simulink model "TopLevel_Turbofan_DT_Faults"  (R2025a)
settings: Solver=ode15s  StartTime=0.0  StopTime=500  MaxStep=0.01  RelTol=1e-3
undefined symbols (not defined in the file or in its folder): BPR_design, DoUpgrade, Eff_hpt_map, Eff_Mod_Fan, Eff_Mod_HPC, Eff_Mod_HPC_Up, Eff_Mod_HPT, Eff_Mod_HPT_Up, Eff_Mod_LPC, Eff_Mod_LPC_Up, Eff_Mod_LPT, eta_hpc_map, eta_lpc_map, eta_lpt_map, Fan_eta_data, Fan_PR_data, FaultMode, flow_vec_fan, norm_flow_hpt, norm_speed_hpt, PR_hpc_map, PR_lpc_map, PR_lpt_map, speed_vec_fan, speed_vec_hpc, speed_vec_lpc, speed_vec_lpt, Torque_hpt_map, Wc_hpc_bp, Wc_lpc_bp, Wc_lpt_bp
libraries: fl_lib x10, nesl_utility x10, simulink x2, sdl_lib x2
(part 1 of 2)
settings Model: Creator=ramch  LastModifiedBy=ramch
settings DataIOCC: SaveFormat=StructureWithTime  SaveOutput=off  SaveState=on  DSMLogging=off  SaveTime=off  ReturnWorkspaceOutputs=off
settings SimscapeCC: SimscapeLogType=all  SimscapeLogSimulationStatistics=on  SimscapeLogToSDI=on  SimscapeLogOpenViewer=on  SimscapeLogName=simlog_TopLevel_Turbofan_DT_PDM  SimscapeLogLimitData=off

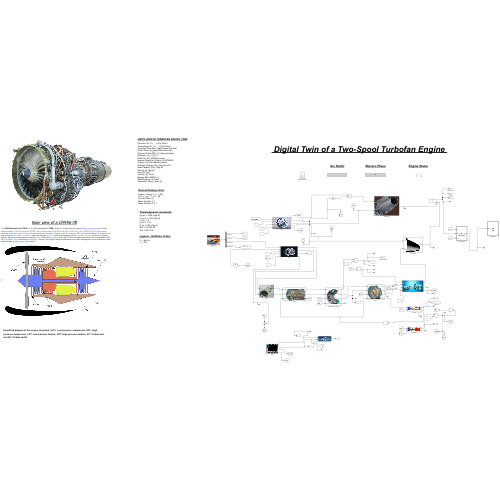
[thumbnail: Simulink's stored preview of the top-level diagram]
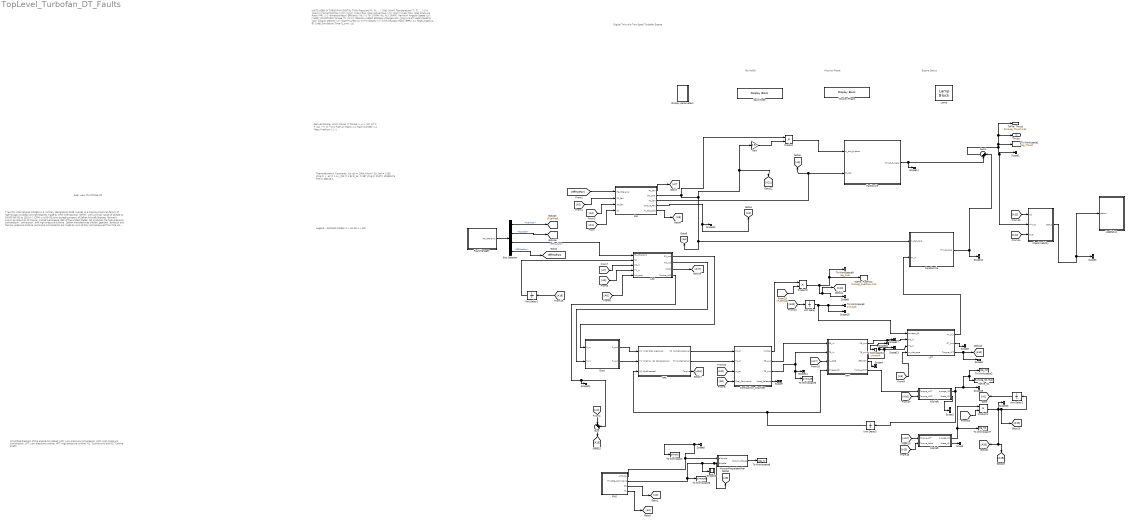
== system TopLevel_Turbofan_DT_Faults ==
  note: UNITS USED IN TURBOFAN DIGITAL TWIN
      | Pressure (P₀, P₁, …): [Pa] (N/m²)
      | Temperature (T₀, T₁, …): [K] (Kelvin)
      | Corrected Flow (Wc): [kg/s] (mass flow rate)
      | Actual Flow (ṁ): [kg/s] (mass flow rate)
      | Pressure Ratio (PR): [–] (dimensionless)
      | Efficiency (η): [–] (0–1)
      | RPM (N₁, N₂): [RPM] (rev/min)
      | Angular Speed (ω): [rad/s] (2π·RPM/60)
      | Torque (τ): [N·m] (Newton-meter)
      | Enthalpy Change (Δh): [J/kg] (cp·ΔT)
      | Heat Capacity (Cp): [J/kg·K]
      | Density (ρ): [kg/m³]
      | Area (A): [m²]
      | Velocity (V): [m/s]
      | Bypass Ratio (BPR): [–]
      | Shaft Angle (φ, θ): [rad]
      | Simulation Time (t_sim): [s]
  note: Digital Twin of a Two-Spool Turbofan Engine
  note: Engine Status
  note: Simplified diagram of the engine simulated (LPC: Low pressure compressor, HPC: High pressure compressor, LPT: Low pressure turbine, HPT: High pressure turbine, N1: Turbine axis and N2: Turbine shaft).
  note: T he CFM International CFM56 (U.S. military designation F108 ) series is a Franco-American family of high-bypass turbofan aircraft engines made by CFM International (CFMI), with a thrust range of 18,500 to 34,000 lbf (82 to 150 kN ). CFMI is a 50–50 joint-owned company of Safran Aircraft Engines (formerly known as Snecma) of France, and GE Aerospace (GE) of the United States. GE produces the high-pressure compressor , combustor , and high-pressure turbine , Safran manufactures the fan, gearbox , exhaust and the low-pressure turbine, and some components are made by Avio of Italy and Honeywell from the US. Both companies have their own final assembly line, GE in Evendale, Ohio , and Safran in Villaroche , France. The engine initially had extremely slow sales but has gone on to become the most used turbofan aircraft engine in the world.
  note: Legend – Go/NoGo Codes:
      |
      | 0 → No Go
      | 1 → GO
  note: Rear view of a CFM56-7B
  note: Derived Display Units:
      | Power = Torque × ω → [W]
      | ΔT = T_out − T_in → [K]
      | Fuel-Air Ratio: [–]
      | Mach Number: [–]
      | Mass Fraction X: [–]
  note: Go/ NoGO
  note: Thermodynamic Constants:
      | Cp_air = 1004 J/(kg·K)
      | Cp_hot = 1150 J/(kg·K)
      | γ_air = 1.4
      | γ_hot = 1.33
      | R_air = 287 J/(kg·K)
      | Pref = 101325 Pa
      | Tref = 288.15 K
  note: Mission Phase
  Bus Selector : BusSelector  OutputSignals=FuelMod,N1Scale,EffModLPC,EffModFan
  CheckViability : MATLAB Function  TreatAsAtomicUnit=on
  Combustion_Chamber : Subsystem
      mask Display: image('CC.jpg');
  CoreNozzle : Subsystem
      mask Display: image('CN.jpg');
  Display parameters : Subsystem
  Duct : Subsystem
      mask Display: image('Duct.jpg');
  FMS : Subsystem
      mask Display: image('FMS.jpg');
  Fan : Subsystem
      mask Display: image('Fan.jpg');
  FanNozzle : Subsystem
      mask Display: image('FN.jpg');
  FaultManager : Subsystem
      mask Display: image('Fault.jpg');
  Gain : Gain  Gain=5.5
  HPC : Subsystem
      mask Display: image('HPC.jpg');
  HPT : Subsystem
      mask Display: image('HPT.jpg');
  LPC : Subsystem
      mask Display: image('LPC.png');
  LPT : Subsystem
      mask Display: image('LPT.jpg');
  Lamp : LampBlock  LabelPosition=Hide  DefaultColor=[192.0, 192.0, 192.0]  Icon=CheckEngine
  LogStatus : MATLAB Function  TreatAsAtomicUnit=on
  Mission Phase : DisplayBlock  LabelPosition=Hide  Transparency=1  GridColor=[0.502, 0.502, 0.502]
  MissionPhaseIdentifier : Subsystem
      mask Display: image('Mission.jpg');
  N1shaft : Subsystem
      mask Display: image('shaft.jpg');
  N2shaft : Subsystem
      mask Display: image('shaft.jpg');
  Product : Product
  Product1 : Product
  Product2 : Product
  Scope{,1..21} (22 alike) : Scope
      Scope settings: ActiveDisplayYMinimum=-1  ActiveDisplayYMaximum=1
      Scope1 settings: ActiveDisplayYMinimum=-1  ActiveDisplayYMaximum=1
      Scope10 settings: ActiveDisplayYMinimum=-0.45859345963387366  ActiveDisplayYMaximum=1.635778226221027  DataLoggingVariableName=ScopeData10
      Scope11 settings: ActiveDisplayYMinimum=-1  ActiveDisplayYMaximum=1  DataLoggingVariableName=ScopeData11
      Scope12 settings: ActiveDisplayYMinimum=-1  ActiveDisplayYMaximum=1  DataLoggingVariableName=ScopeData12
      Scope13 settings: ActiveDisplayYMinimum=-609.11434420859632  ActiveDisplayYMaximum=1781.0190470175871  DataLoggingVariableName=ScopeData13
      Scope14 settings: ActiveDisplayYMinimum=-1  ActiveDisplayYMaximum=1  DataLoggingVariableName=ScopeData14
      Scope15 settings: ActiveDisplayYMinimum=-1  ActiveDisplayYMaximum=1  DataLoggingVariableName=ScopeData15
      Scope16 settings: ActiveDisplayYMinimum=-4.3963021341582635  ActiveDisplayYMaximum=4.6281003390981308  DataLoggingVariableName=ScopeData16
      Scope17 settings: ActiveDisplayYMinimum=-2.2429279816897957E+23  ActiveDisplayYMaximum=2.0186351835208165E+24  DataLoggingVariableName=ScopeData17
      Scope18 settings: ActiveDisplayYMinimum=-513.71209028734575  ActiveDisplayYMaximum=1737.7811833983071  DataLoggingVariableName=ScopeData18
      Scope19 settings: ActiveDisplayYMinimum=-0.12499999999999997  ActiveDisplayYMaximum=1.125  DataLoggingVariableName=ScopeData19
      Scope2 settings: ActiveDisplayYMinimum=-1  ActiveDisplayYMaximum=1  DataLoggingVariableName=ScopeData2
      Scope20 settings: ActiveDisplayYMinimum=-3.6198875871994079E+21  ActiveDisplayYMaximum=5.5031192284267649E+20  DataLoggingVariableName=ScopeData20
      Scope21 settings: ActiveDisplayYMinimum=-0.23453341351778778  ActiveDisplayYMaximum=0.2421108240195578  DataLoggingVariableName=ScopeData21
      Scope3 settings: ActiveDisplayYMinimum=-1  ActiveDisplayYMaximum=1  DataLoggingVariableName=ScopeData3
      Scope4 settings: ActiveDisplayYMinimum=-1.4197628335321743E+18  ActiveDisplayYMaximum=1.5775142594801933E+17  DataLoggingVariableName=ScopeData4
      Scope5 settings: ActiveDisplayYMinimum=-5201.9747686683695  ActiveDisplayYMaximum=12688.378863465885  DataLoggingVariableName=ScopeData5
      Scope6 settings: ActiveDisplayYMinimum=-1  ActiveDisplayYMaximum=1  DataLoggingVariableName=ScopeData6
      Scope7 settings: ActiveDisplayYMinimum=952444.62242727727  ActiveDisplayYMaximum=9.2631053030945715E+6  DataLoggingVariableName=ScopeData7
      Scope8 settings: ActiveDisplayYMinimum=-1  ActiveDisplayYMaximum=1  DataLoggingVariableName=ScopeData8
      Scope9 settings: ActiveDisplayYMinimum=-1  ActiveDisplayYMaximum=1  DataLoggingVariableName=ScopeData9
  Sum : Sum  Inputs=|++
  Sum1 : Sum  Inputs=|++
  To Workspace : ToWorkspace  VariableName=simout  SaveFormat=Timeseries  SampleTime=-1
  To Workspace1 : ToWorkspace  VariableName=log_Thrust  SaveFormat=Timeseries  SampleTime=-1
  To Workspace2 : ToWorkspace  VariableName=log_N2  SaveFormat=Timeseries  SampleTime=-1
  To Workspace3 : ToWorkspace  VariableName=simout3  SaveFormat=Timeseries  SampleTime=-1
  To Workspace4 : ToWorkspace  VariableName=simout4  SaveFormat=Timeseries  SampleTime=-1
  To Workspace5 : ToWorkspace  VariableName=simout5  SaveFormat=Timeseries  SampleTime=-1
  To Workspace6 : ToWorkspace  VariableName=simout6  SaveFormat=Timeseries  SampleTime=-1
  To Workspace7 : ToWorkspace  VariableName=log_N1  SaveFormat=Timeseries  SampleTime=-1
  To Workspace8 : ToWorkspace  VariableName=log_N  SaveFormat=Timeseries  SampleTime=-1
  To Workspace9 : ToWorkspace  VariableName=log_Fuel  SaveFormat=Timeseries  SampleTime=-1
  ToFile_FuelFlow : ToFile  Filename=RunLog_FuelFlow.mat  MatrixName=m_fuel  SaveFormat=Timeseries
  ToFile_N1 : ToFile  Filename=RunLog_N1.mat  MatrixName=omega_N1
  ToFile_Thrust : ToFile  Filename=RunLog_Thrust.mat  MatrixName=Thrust
  Unit Delay{,1..3} (4 alike) : UnitDelay  InitialCondition=1  SampleTime=-1  HasFrameUpgradeWarning=on
  fault Mode : DisplayBlock  LabelPosition=Hide  Transparency=1  GridColor=[0.502, 0.502, 0.502]
  Thrust : Outport
  wires:
  N2shaft/2(theta_N2) -> Scope1/1
  FaultManager/1(FaultParams) -> Bus Selector/1
  [A7] -> LPC/3(P2_in)
  Product1/1 -> [A20], [A18], [A13], Unit Delay2/1, Scope16/1
  HPC/1(P2 (outlet pressure)) -> Combustion_Chamber/1(P4_in)
  Fan/3(T1_fan) -> [A5], FanNozzle/2(T1_fan)
  CoreNozzle/1(Thrust_core) -> Scope12/1, Sum1/1
  Product2/1 -> To Workspace9/1, ToFile_FuelFlow/1, Scope8/1, [A14]
  Bus Selector/3 -> LPC/1(FaultParams)  "<EffModLPC>"
  Product/1 -> FanNozzle/1(m_dot_bypass)
  LPC/1(P3_out) -> Duct/1(P_in)
  Duct/2(T_out) -> HPC/2("T1 (inlet total temperature) ")
  Bus Selector/4 -> [EffModFan]  "<EffModFan>"
  [A6] -> LPC/5(Wc_core)
  [A4] -> Sum/1
  LPC/2(T3_out) -> Duct/2(T_in)
  HPC/2(T2 (outlet temp)) -> Combustion_Chamber/2(T4_in)
  LPC/4(Torque_LPC) -> Sum/2, Scope21/1
  N2shaft/1(omega_N2) -> To Workspace2/1, ToFile_N1/1, Scope15/1, Unit Delay3/1
  [EffModFan] -> Fan/1(FaultParams)
  Gain/1 -> Product/2
  [A2] -> Fan/2(P0_fan)
  [A3] -> Fan/3(T0_fan)
  [A1] -> Fan/4(N1)
  Duct/1(P_out) -> HPC/1(P1 (inlet total pressure))
  HPT/2(T6_out) -> Scope18/1, To Workspace4/1, Scope13/1, LPT/3(T6_in)
  Fan/1(" P1_fan") -> [A7]
  Fan/5(m_dot_core) -> [A9]
  HPT/1(P6_out) -> LPT/2(P6_in), Scope17/1
  FMS/1(Altitude) -> To Workspace/1, Scope5/1, MissionPhaseIdentifier/1(altitude)
  FMS/2(Throttle_Command) -> [A8], MissionPhaseIdentifier/2(throttle), Scope10/1, To Workspace6/1
  FMS/3(P0) -> [A2]
  FMS/4(T0) -> [A3]
  LPT/3(Torque_LPT) -> Scope9/1, [A10]
  Combustion_Chamber/2(P5_out) -> HPT/1(P5_in)
  Unit Delay3/1 -> HPC/3(N2 (shaft speed)), HPT/4(omega_N2)
  Combustion_Chamber/4(Heat_Release) -> Scope7/1
  Combustion_Chamber/3(T5_out) -> HPT/2(T5_in), To Workspace5/1, Scope14/1
  Combustion_Chamber/1(m_fuel) -> Product2/1
  MissionPhaseIdentifier/1(Mission_Phase) -> To Workspace8/1
  Unit Delay/1 -> Scope19/1, To Workspace3/1, LPT/1(omega_N1)
  Sum1/1 -> ToFile_Thrust/1, Thrust/1, To Workspace1/1, CheckViability/2(Thrust), Scope2/1
  HPT/4(Torque_HPT) -> N2shaft/1(Torque_HPT)
  FanNozzle/1(Thrust_bypass) -> Sum1/2, Scope11/1
  HPT/3(Eff_HPT) -> Scope4/1
  [A9] -> LPT/4(m_dot_core)
  LPT/2(P7_out) -> Scope6/1
  LPT/1(T7_out) -> CoreNozzle/2(T7_in)
  Unit Delay2/1 -> [A1]
  N1shaft/1(omega_N1) -> Product1/1, To Workspace7/1
  N1shaft/2(theta_N1) -> Scope/1
  CheckViability/1(status) -> Scope3/1, LogStatus/1(status)
  Fan/4(Torque_Fan) -> [A4], Scope20/1
  Fan/2(Wc_core) -> CoreNozzle/1(m_dot_core), [A6], [A21], Gain/1, Product/1
  [A13] -> CheckViability/1(N1)
  [A14] -> CheckViability/3(Fuel)
  Sum/1 -> [A15]
  [A15] -> N1shaft/2(Torque_Load)
  Bus Selector/2 -> [N1Scale]  "<N1Scale>"
  [N1Scale] -> Product1/2
  HPC/3(Torque) -> [A16]
  [A16] -> N2shaft/2(Torque_HPC)
  LPC/3(mdot) -> [A17]
  [A17] -> HPT/3(m_dot5)
  [A18] -> Unit Delay1/1
  Unit Delay1/1 -> LPC/2(N1)
  [A20] -> Unit Delay/1
  [A21] -> Combustion_Chamber/3(m_air)
  Bus Selector/1 -> [FuelMod]  "<FuelMod>"
  [FuelMod] -> Product2/2
  [A5] -> LPC/4(T2_in)
  [A8] -> Combustion_Chamber/4(Fuel_Command)
  [A10] -> N1shaft/1(Torque_LPT)

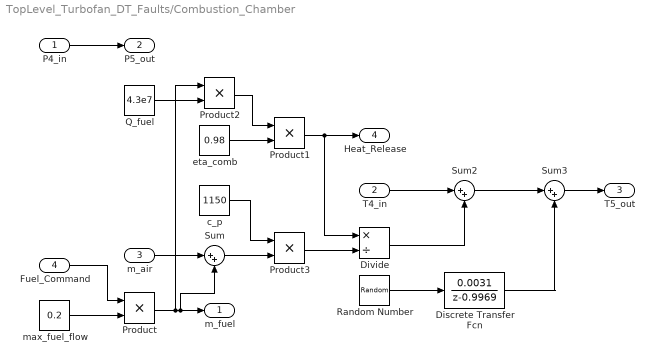
== system TopLevel_Turbofan_DT_Faults/Combustion_Chamber ==
  P4_in : Inport
  T4_in : Inport  Port=2
  m_air : Inport  Port=3
  Fuel_Command : Inport  Port=4
  Discrete Transfer Fcn : DiscreteTransferFcn  Numerator=0.0031  Denominator=1 -0.9969  InitialStates=0.001
  Divide : Product  Inputs=*/
  Product{,1..3} (4 alike) : Product
  Q_fuel : Constant  Value=4.3e7
  Random Number : RandomNumber  Variance=0.5  SampleTime=0.001
  Sum : Sum  Inputs=|++
  Sum2 : Sum  Inputs=|++
  Sum3 : Sum  Inputs=|++
  c_p : Constant  Value=1150
  eta_comb : Constant  Value=0.98
  max_fuel_flow : Constant  Value=0.2
  m_fuel : Outport
  P5_out : Outport  Port=2
  T5_out : Outport  Port=3
  Heat_Release : Outport  Port=4
  wires:
  T4_in/1 -> Sum2/1
  P4_in/1 -> P5_out/1
  Fuel_Command/1 -> Product/1
  m_air/1 -> Sum/1
  Sum3/1 -> T5_out/1
  Sum2/1 -> Sum3/1
  Sum/1 -> Product3/2
  eta_comb/1 -> Product1/2
  c_p/1 -> Product3/1
  max_fuel_flow/1 -> Product/2
  Random Number/1 -> Discrete Transfer Fcn/1
  Product3/1 -> Divide/2
  Product1/1 -> Divide/1, Heat_Release/1
  Product2/1 -> Product1/1
  Q_fuel/1 -> Product2/2
  Divide/1 -> Sum2/2
  Product/1 -> Sum/2, m_fuel/1, Product2/1
  Discrete Transfer Fcn/1 -> Sum3/2

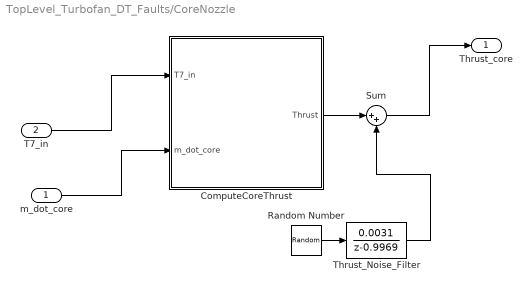
== system TopLevel_Turbofan_DT_Faults/CoreNozzle ==
  m_dot_core : Inport
  T7_in : Inport  Port=2
  ComputeCoreThrust : MATLAB Function  TreatAsAtomicUnit=on
  Random Number : RandomNumber  Variance=500  SampleTime=0.001
  Sum : Sum  Inputs=|++
  Thrust_Noise_Filter : DiscreteTransferFcn  Numerator=0.0031  Denominator=1 -0.9969  InitialStates=0.001
  Thrust_core : Outport
  wires:
  Sum/1 -> Thrust_core/1
  T7_in/1 -> ComputeCoreThrust/1(T7_in)
  Random Number/1 -> Thrust_Noise_Filter/1
  m_dot_core/1 -> ComputeCoreThrust/2(m_dot_core)
  ComputeCoreThrust/1(Thrust) -> Sum/1
  Thrust_Noise_Filter/1 -> Sum/2

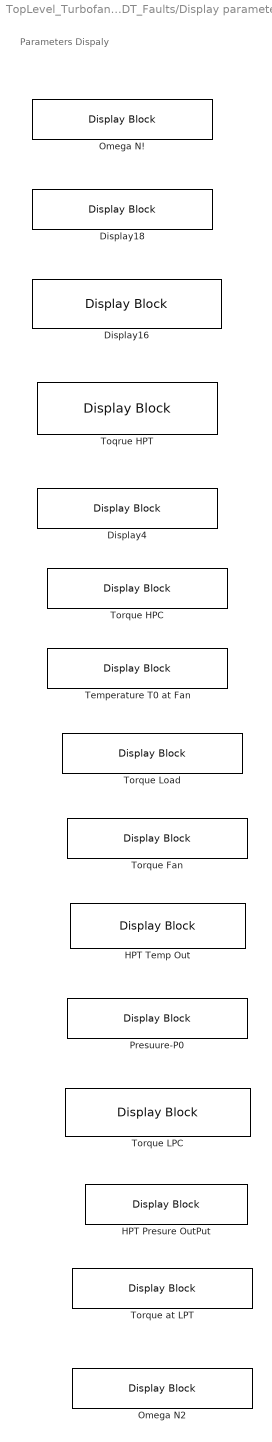
== system TopLevel_Turbofan_DT_Faults/Display parameters ==
  note: Parameters Dispaly
  Display16 : DisplayBlock  LabelPosition=Hide  Transparency=1  GridColor=[0.502, 0.502, 0.502]
  Display18 : DisplayBlock  LabelPosition=Hide  Transparency=1  GridColor=[0.502, 0.502, 0.502]
  Display4 : DisplayBlock  LabelPosition=Hide  Transparency=1  GridColor=[0.502, 0.502, 0.502]
  HPT Presure OutPut : DisplayBlock  LabelPosition=Hide  Transparency=1  GridColor=[0.502, 0.502, 0.502]
  HPT Temp Out : DisplayBlock  LabelPosition=Hide  Transparency=1  GridColor=[0.502, 0.502, 0.502]
  Omega N! : DisplayBlock  LabelPosition=Hide  Transparency=1  GridColor=[0.502, 0.502, 0.502]
  Omega N2 : DisplayBlock  LabelPosition=Hide  Transparency=1  GridColor=[0.502, 0.502, 0.502]
  Presuure-P0 : DisplayBlock  LabelPosition=Hide  Transparency=1  GridColor=[0.502, 0.502, 0.502]
  Temperature T0 at Fan : DisplayBlock  LabelPosition=Hide  Transparency=1  GridColor=[0.502, 0.502, 0.502]
  Toqrue HPT : DisplayBlock  LabelPosition=Hide  Transparency=1  GridColor=[0.502, 0.502, 0.502]
  Torque Fan : DisplayBlock  LabelPosition=Hide  Transparency=1  GridColor=[0.502, 0.502, 0.502]
  Torque HPC : DisplayBlock  LabelPosition=Hide  Transparency=1  GridColor=[0.502, 0.502, 0.502]
  Torque LPC : DisplayBlock  LabelPosition=Hide  Transparency=1  GridColor=[0.502, 0.502, 0.502]
  Torque Load : DisplayBlock  LabelPosition=Hide  Transparency=1  GridColor=[0.502, 0.502, 0.502]
  Torque at LPT : DisplayBlock  LabelPosition=Hide  Transparency=1  GridColor=[0.502, 0.502, 0.502]

== system TopLevel_Turbofan_DT_Faults/Duct ==
  P_in : Inport
  T_in : Inport  Port=2
  Gain : Gain  Gain=0.98
  P_out : Outport
  T_out : Outport  Port=2
  wires:
  Gain/1 -> P_out/1
  T_in/1 -> T_out/1
  P_in/1 -> Gain/1

== system TopLevel_Turbofan_DT_Faults/FMS ==
  Altitude_Profile : simulink/Sources/Repeating Sequence Interpolated  OutValues=[0 1500 6000 10000 10000 5000 0]  TimeValues=[0 50 100 200 300 400 500]  LookUpMeth=Interpolation-Use End Values  tsamp=0.1  OutMin=[]  OutMax=[]  OutDataTypeStr=double  OutputDataTypeScalingMode=double  OutDataType=fixdt(0,8)  OutScaling=2^-10
  AtmosphereModel : MATLAB Function  TreatAsAtomicUnit=on
  Throttle_Command_Profile : simulink/Sources/Repeating Sequence Interpolated  OutValues=[1.0 0.9 0.7 0.5 0.5 0.6 0.3]  TimeValues=[0 50 100 200 300 400 500]  LookUpMeth=Use Input Below  tsamp=0.1  OutMin=[]  OutMax=[]  OutDataTypeStr=double  OutputDataTypeScalingMode=double  OutDataType=fixdt(0,8)  OutScaling=2^-10
  Altitude : Outport
  Throttle_Command : Outport  Port=2
  P0 : Outport  Port=3
  T0 : Outport  Port=4
  wires:
  AtmosphereModel/1(P0) -> P0/1
  AtmosphereModel/2(T0) -> T0/1
  Altitude_Profile/1 -> AtmosphereModel/1(Altitude), Altitude/1
  Throttle_Command_Profile/1 -> Throttle_Command/1

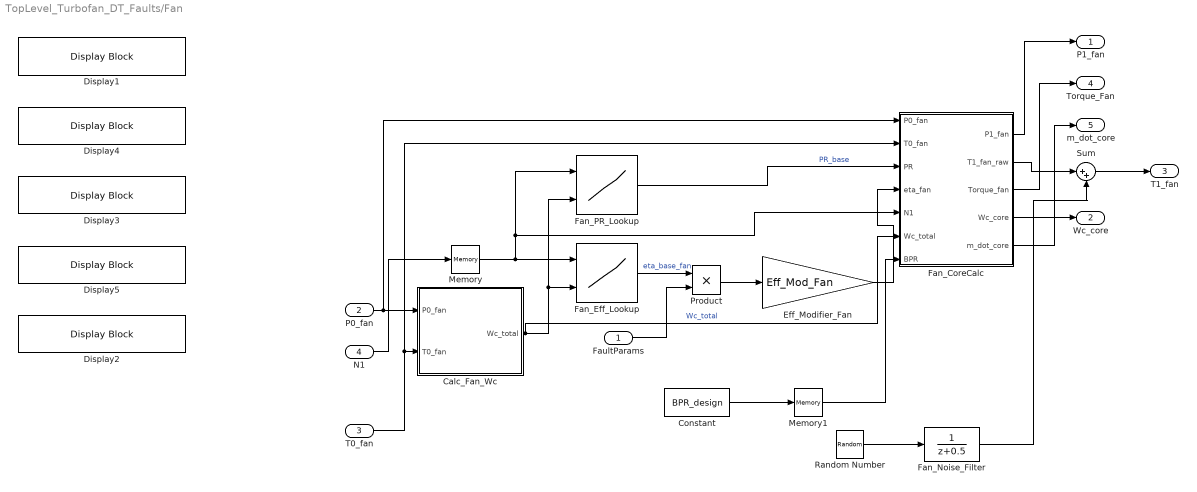
== system TopLevel_Turbofan_DT_Faults/Fan ==
  FaultParams : Inport
  P0_fan : Inport  Port=2
  T0_fan : Inport  Port=3
  N1 : Inport  Port=4
  Calc_Fan_Wc : MATLAB Function  TreatAsAtomicUnit=on
  Constant : Constant  Value=BPR_design
  Display{1..5} (5 alike) : DisplayBlock  LabelPosition=Hide  Transparency=1  GridColor=[0.502, 0.502, 0.502]
  Eff_Modifier_Fan : Gain  Gain=Eff_Mod_Fan
  Fan_CoreCalc : MATLAB Function  TreatAsAtomicUnit=on
  Fan_Eff_Lookup : Lookup_n-D  BreakpointsForDimension1=speed_vec_fan  BreakpointsForDimension2=flow_vec_fan  Table=Fan_eta_data  ExtrapMethod=Clip  InternalRulePriority=Speed  RndMeth=Simplest
      settings: InputPortMap=u0,u1
  Fan_Noise_Filter : DiscreteTransferFcn
  Fan_PR_Lookup : Lookup_n-D  BreakpointsForDimension1=speed_vec_fan  BreakpointsForDimension2=flow_vec_fan  Table=Fan_PR_data  ExtrapMethod=Clip  InternalRulePriority=Speed  RndMeth=Simplest
      settings: InputPortMap=u0,u1
  Memory : Memory
  Memory1 : Memory
  Product : Product
  Random Number : RandomNumber  Variance=(0.5)  SampleTime=0.001
  Sum : Sum  Inputs=|++
  " P1_fan" : Outport
  Wc_core : Outport  Port=2
  T1_fan : Outport  Port=3
  Torque_Fan : Outport  Port=4
  m_dot_core : Outport  Port=5
  wires:
  FaultParams/1 -> Product/2
  T0_fan/1 -> Fan_CoreCalc/2(T0_fan), Calc_Fan_Wc/2(T0_fan)
  Calc_Fan_Wc/1(Wc_total) -> Fan_Eff_Lookup/2, Fan_PR_Lookup/2, Fan_CoreCalc/6(Wc_total)  "Wc_total"
  N1/1 -> Memory/1
  P0_fan/1 -> Fan_CoreCalc/1(P0_fan), Calc_Fan_Wc/1(P0_fan)
  Memory/1 -> Fan_CoreCalc/5(N1), Fan_PR_Lookup/1, Fan_Eff_Lookup/1
  Fan_Eff_Lookup/1 -> Product/1  "eta_base_fan"
  Fan_PR_Lookup/1 -> Fan_CoreCalc/3(PR)  "PR_base"
  Product/1 -> Eff_Modifier_Fan/1
  Eff_Modifier_Fan/1 -> Fan_CoreCalc/4(eta_fan)
  Constant/1 -> Memory1/1
  Memory1/1 -> Fan_CoreCalc/7(BPR)
  Random Number/1 -> Fan_Noise_Filter/1
  Fan_CoreCalc/1(P1_fan) -> " P1_fan"/1
  Fan_CoreCalc/2(T1_fan_raw) -> Sum/1
  Fan_CoreCalc/3(Torque_fan) -> Torque_Fan/1
  Fan_CoreCalc/4(Wc_core) -> Wc_core/1
  Fan_CoreCalc/5(m_dot_core) -> m_dot_core/1
  Fan_Noise_Filter/1 -> Sum/2
  Sum/1 -> T1_fan/1

== system TopLevel_Turbofan_DT_Faults/FanNozzle ==
  m_dot_bypass : Inport
  T1_fan : Inport  Port=2
  ComputeCoreThrust : MATLAB Function  TreatAsAtomicUnit=on
  Random Number : RandomNumber  Variance=200  SampleTime=0.001
  Sum : Sum  Inputs=|++
  Thrust_Noise_Filter : DiscreteTransferFcn  Numerator=0.0031  Denominator=1 -0.9969  InitialStates=0.001
  Thrust_bypass : Outport
  wires:
  T1_fan/1 -> ComputeCoreThrust/1(T1_fan)
  Random Number/1 -> Thrust_Noise_Filter/1
  Sum/1 -> Thrust_bypass/1
  Thrust_Noise_Filter/1 -> Sum/2
  ComputeCoreThrust/1(Thrust) -> Sum/1
  m_dot_bypass/1 -> ComputeCoreThrust/2(m_dot_bypass)

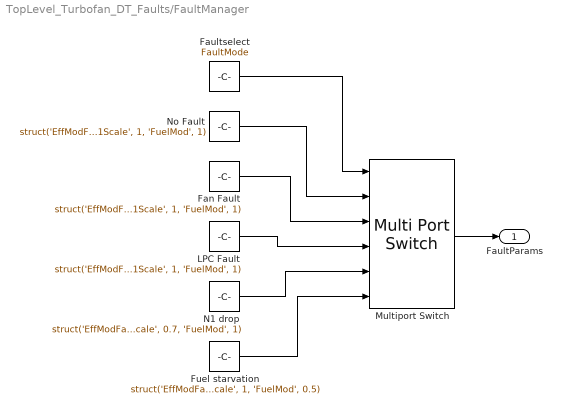
== system TopLevel_Turbofan_DT_Faults/FaultManager ==
  " N1 drop" : Constant  Value=struct('EffModFan', 1, 'EffModLPC', 1, 'N1Scale', 0.7, 'FuelMod', 1)  OutDataTypeStr=Bus: FaultParamsBus
  Fan Fault : Constant  Value=struct('EffModFan', 0.6, 'EffModLPC', 1, 'N1Scale', 1, 'FuelMod', 1)  OutDataTypeStr=Bus: FaultParamsBus
  Faultselect : Constant  Value=FaultMode
  Fuel starvation : Constant  Value=struct('EffModFan', 1, 'EffModLPC', 1, 'N1Scale', 1, 'FuelMod', 0.5)  OutDataTypeStr=Bus: FaultParamsBus
  LPC Fault : Constant  Value=struct('EffModFan', 1, 'EffModLPC', 0.5, 'N1Scale', 1, 'FuelMod', 1)  OutDataTypeStr=Bus: FaultParamsBus
  Multiport Switch : MultiPortSwitch  DataPortOrder=Zero-based contiguous  Inputs=5  zeroidx=on  SaturateOnIntegerOverflow=off  InputSameDT=off
  No Fault : Constant  Value=struct('EffModFan', 1, 'EffModLPC', 1, 'N1Scale', 1, 'FuelMod', 1)  OutDataTypeStr=Bus: FaultParamsBus
  FaultParams : Outport
  wires:
  No Fault/1 -> Multiport Switch/2
  Fan Fault/1 -> Multiport Switch/3
  LPC Fault/1 -> Multiport Switch/4
  " N1 drop"/1 -> Multiport Switch/5
  Fuel starvation/1 -> Multiport Switch/6
  Multiport Switch/1 -> FaultParams/1
  Faultselect/1 -> Multiport Switch/1

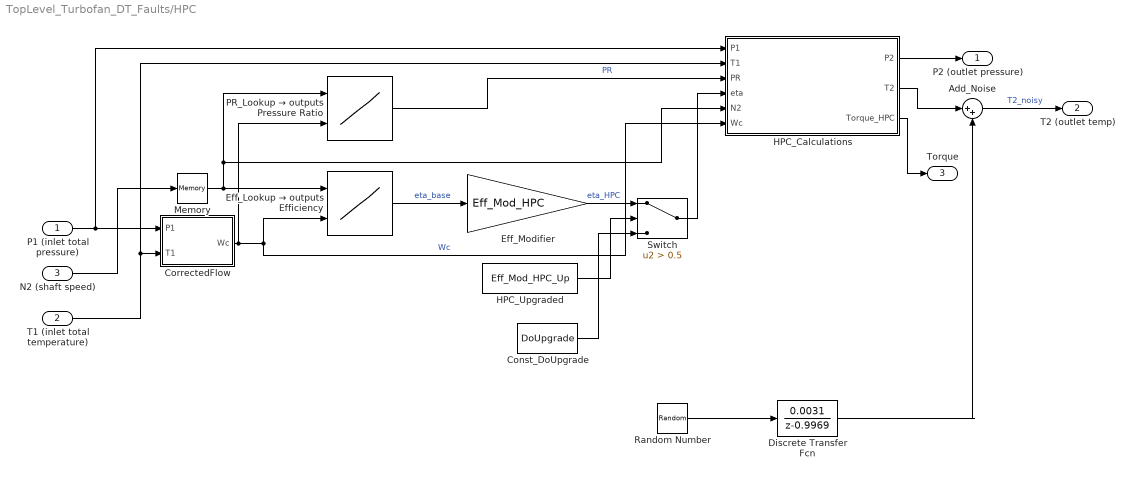
== system TopLevel_Turbofan_DT_Faults/HPC ==
  P1 (inlet total pressure) : Inport
  "T1 (inlet total temperature) " : Inport  Port=2
  N2 (shaft speed) : Inport  Port=3
  Add_Noise : Sum  Inputs=|++
  Const_DoUpgrade : Constant  Value=DoUpgrade  SampleTime=-1
  CorrectedFlow : MATLAB Function  TreatAsAtomicUnit=on
  Discrete Transfer Fcn : DiscreteTransferFcn  Numerator=0.0031  Denominator=1 -0.9969  InitialStates=0.001
  Eff_Lookup → outputs Efficiency : Lookup_n-D  BreakpointsForDimension1=speed_vec_hpc  BreakpointsForDimension2=Wc_hpc_bp  Table=eta_hpc_map  InternalRulePriority=Speed  RndMeth=Simplest
      settings: InputPortMap=u0,u1
  Eff_Modifier : Gain  Gain=Eff_Mod_HPC
  HPC_Calculations : MATLAB Function  TreatAsAtomicUnit=on
  HPC_Upgraded : Constant  Value=Eff_Mod_HPC_Up
  Memory : Memory
  PR_Lookup → outputs Pressure Ratio : Lookup_n-D  BreakpointsForDimension1=speed_vec_hpc  BreakpointsForDimension2=Wc_hpc_bp  Table=PR_hpc_map  InternalRulePriority=Speed  RndMeth=Simplest
      settings: InputPortMap=u0,u1
  Random Number : RandomNumber  Variance=(0.5)  SampleTime=0.001
  Switch : Switch  Criteria=u2 > Threshold  Threshold=0.5  SaturateOnIntegerOverflow=off  InputSameDT=off
  P2 (outlet pressure) : Outport
  T2 (outlet temp) : Outport  Port=2
  Torque : Outport  Port=3
  wires:
  Const_DoUpgrade/1 -> Switch/3
  "T1 (inlet total temperature) "/1 -> HPC_Calculations/2(T1), CorrectedFlow/2(T1)
  N2 (shaft speed)/1 -> Memory/1
  Add_Noise/1 -> T2 (outlet temp)/1  "T2_noisy"
  P1 (inlet total pressure)/1 -> HPC_Calculations/1(P1), CorrectedFlow/1(P1)
  Memory/1 -> HPC_Calculations/5(N2), PR_Lookup → outputs Pressure Ratio/1, Eff_Lookup → outputs Efficiency/1
  Eff_Lookup → outputs Efficiency/1 -> Eff_Modifier/1  "eta_base"
  Discrete Transfer Fcn/1 -> Add_Noise/2
  CorrectedFlow/1(Wc) -> HPC_Calculations/6(Wc), Eff_Lookup → outputs Efficiency/2, PR_Lookup → outputs Pressure Ratio/2  "Wc"
  PR_Lookup → outputs Pressure Ratio/1 -> HPC_Calculations/3(PR)  "PR"
  HPC_Calculations/1(P2) -> P2 (outlet pressure)/1
  Eff_Modifier/1 -> Switch/1  "eta_HPC"
  HPC_Upgraded/1 -> Switch/2
  Switch/1 -> HPC_Calculations/4(eta)
  Random Number/1 -> Discrete Transfer Fcn/1
  HPC_Calculations/2(T2) -> Add_Noise/1
  HPC_Calculations/3(Torque_HPC) -> Torque/1

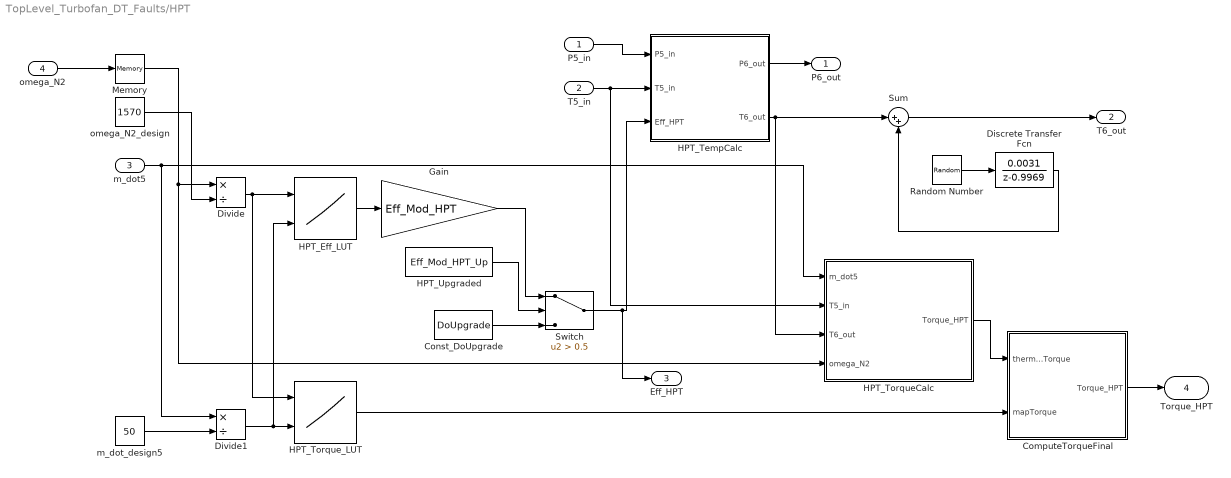
== system TopLevel_Turbofan_DT_Faults/HPT ==
  P5_in : Inport
  T5_in : Inport  Port=2
  m_dot5 : Inport  Port=3
  omega_N2 : Inport  Port=4
  ComputeTorqueFinal : MATLAB Function  TreatAsAtomicUnit=on
  Const_DoUpgrade : Constant  Value=DoUpgrade  SampleTime=-1
  Discrete Transfer Fcn : DiscreteTransferFcn  Numerator=0.0031  Denominator=1 -0.9969  InitialStates=0.001
  Divide : Product  Inputs=*/
  Divide1 : Product  Inputs=*/
  Gain : Gain  Gain=Eff_Mod_HPT
  HPT_Eff_LUT : Lookup_n-D  BreakpointsForDimension1=norm_speed_hpt  BreakpointsForDimension2=norm_flow_hpt  Table=Eff_hpt_map  InternalRulePriority=Speed  RndMeth=Simplest
      settings: InputPortMap=u0,u1
  HPT_TempCalc : MATLAB Function  TreatAsAtomicUnit=on
  HPT_TorqueCalc : MATLAB Function  TreatAsAtomicUnit=on
  HPT_Torque_LUT : Lookup_n-D  BreakpointsForDimension1=norm_speed_hpt  BreakpointsForDimension2=norm_flow_hpt  Table=Torque_hpt_map  InternalRulePriority=Speed  RndMeth=Simplest
      settings: InputPortMap=u0,u1
  HPT_Upgraded : Constant  Value=Eff_Mod_HPT_Up
  Memory : Memory
  Random Number : RandomNumber  Variance=0.5  SampleTime=0.1
  Sum : Sum  Inputs=|++
  Switch : Switch  Criteria=u2 > Threshold  Threshold=0.5  SaturateOnIntegerOverflow=off  InputSameDT=off
  m_dot_design5 : Constant  Value=50
  omega_N2_design : Constant  Value=1570
  P6_out : Outport
  T6_out : Outport  Port=2
  Eff_HPT : Outport  Port=3
  Torque_HPT : Outport  Port=4
  wires:
  m_dot5/1 -> HPT_TorqueCalc/1(m_dot5), Divide1/1
  omega_N2/1 -> Memory/1
  Memory/1 -> HPT_TorqueCalc/4(omega_N2), Divide/1
  m_dot_design5/1 -> Divide1/2
  omega_N2_design/1 -> Divide/2
  Discrete Transfer Fcn/1 -> Sum/2
  HPT_Eff_LUT/1 -> Gain/1
  Divide1/1 -> HPT_Eff_LUT/2, HPT_Torque_LUT/2
  HPT_TempCalc/1(P6_out) -> P6_out/1
  Divide/1 -> HPT_Torque_LUT/1, HPT_Eff_LUT/1
  HPT_Torque_LUT/1 -> ComputeTorqueFinal/2(mapTorque)
  Gain/1 -> Switch/1
  HPT_Upgraded/1 -> Switch/2
  HPT_TempCalc/2(T6_out) -> Sum/1, HPT_TorqueCalc/3(T6_out)
  Const_DoUpgrade/1 -> Switch/3
  Random Number/1 -> Discrete Transfer Fcn/1
  P5_in/1 -> HPT_TempCalc/1(P5_in)
  T5_in/1 -> HPT_TorqueCalc/2(T5_in), HPT_TempCalc/2(T5_in)
  Switch/1 -> HPT_TempCalc/3(Eff_HPT), Eff_HPT/1
  Sum/1 -> T6_out/1
  HPT_TorqueCalc/1(Torque_HPT) -> ComputeTorqueFinal/1(thermoTorque)
  ComputeTorqueFinal/1(Torque_HPT) -> Torque_HPT/1

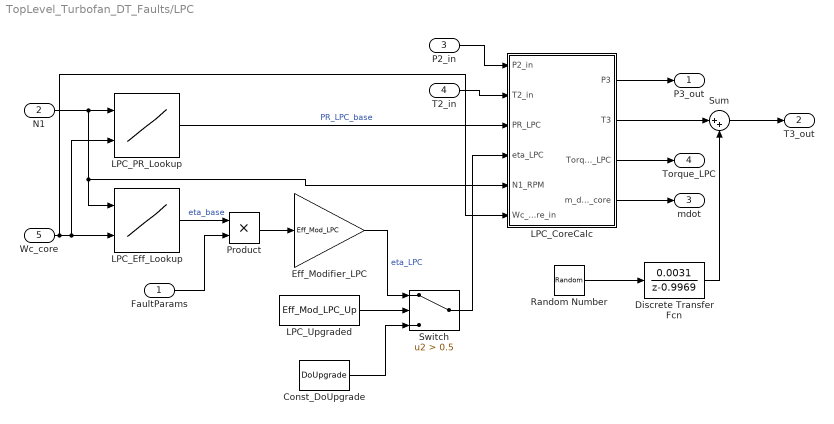
== system TopLevel_Turbofan_DT_Faults/LPC ==
  FaultParams : Inport
  N1 : Inport  Port=2
  P2_in : Inport  Port=3
  T2_in : Inport  Port=4
  Wc_core : Inport  Port=5
  Const_DoUpgrade : Constant  Value=DoUpgrade  SampleTime=-1
  Discrete Transfer Fcn : DiscreteTransferFcn  Numerator=0.0031  Denominator=1 -0.9969  InitialStates=0.001
  Eff_Modifier_LPC : Gain  Gain=Eff_Mod_LPC
  LPC_CoreCalc : MATLAB Function  TreatAsAtomicUnit=on
  LPC_Eff_Lookup : Lookup_n-D  BreakpointsForDimension1=speed_vec_lpc  BreakpointsForDimension2=Wc_lpc_bp  Table=eta_lpc_map  ExtrapMethod=Clip  InternalRulePriority=Speed  RndMeth=Simplest
      settings: InputPortMap=u0,u1
  LPC_PR_Lookup : Lookup_n-D  BreakpointsForDimension1=speed_vec_lpc  BreakpointsForDimension2=Wc_lpc_bp  Table=PR_lpc_map  ExtrapMethod=Clip  InternalRulePriority=Speed  RndMeth=Simplest
      settings: InputPortMap=u0,u1
  LPC_Upgraded : Constant  Value=Eff_Mod_LPC_Up
  Product : Product
  Random Number : RandomNumber  Variance=(0.5)  SampleTime=0.001
  Sum : Sum  Inputs=|++
  Switch : Switch  Criteria=u2 > Threshold  Threshold=0.5  SaturateOnIntegerOverflow=off  InputSameDT=off
  P3_out : Outport
  T3_out : Outport  Port=2
  mdot : Outport  Port=3
  Torque_LPC : Outport  Port=4
  wires:
  Eff_Modifier_LPC/1 -> Switch/1  "eta_LPC"
  LPC_CoreCalc/1(P3) -> P3_out/1
  FaultParams/1 -> Product/2
  Wc_core/1 -> LPC_PR_Lookup/2, LPC_Eff_Lookup/2, LPC_CoreCalc/6(Wc_core_in)
  N1/1 -> LPC_CoreCalc/5(N1_RPM), LPC_Eff_Lookup/1, LPC_PR_Lookup/1
  LPC_Eff_Lookup/1 -> Product/1  "eta_base"
  Switch/1 -> LPC_CoreCalc/4(eta_LPC)
  LPC_PR_Lookup/1 -> LPC_CoreCalc/3(PR_LPC)  "PR_LPC_base"
  LPC_Upgraded/1 -> Switch/2
  Product/1 -> Eff_Modifier_LPC/1
  LPC_CoreCalc/3(Torque_LPC) -> Torque_LPC/1
  Const_DoUpgrade/1 -> Switch/3
  P2_in/1 -> LPC_CoreCalc/1(P2_in)
  T2_in/1 -> LPC_CoreCalc/2(T2_in)
  Random Number/1 -> Discrete Transfer Fcn/1
  LPC_CoreCalc/2(T3) -> Sum/1
  LPC_CoreCalc/4(m_dot_core) -> mdot/1
  Discrete Transfer Fcn/1 -> Sum/2
  Sum/1 -> T3_out/1

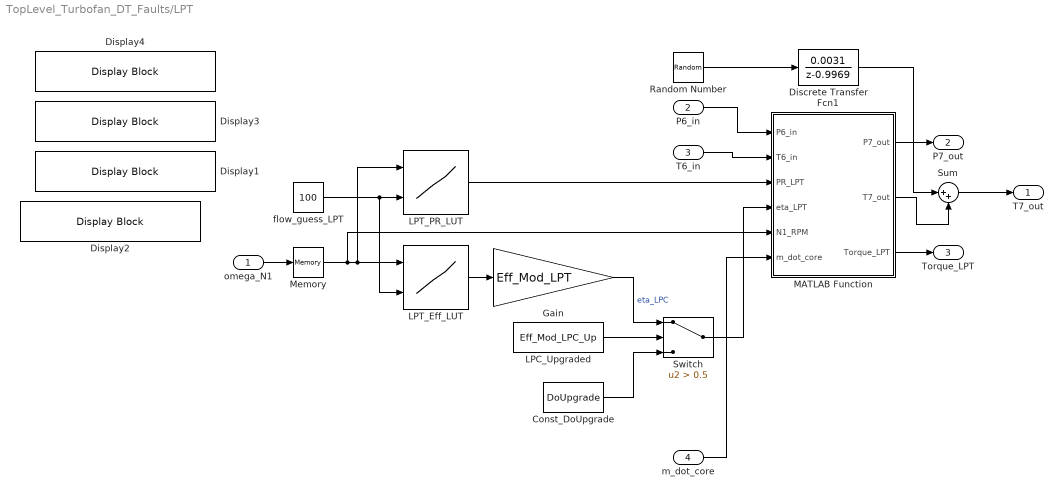
== system TopLevel_Turbofan_DT_Faults/LPT ==
  omega_N1 : Inport
  P6_in : Inport  Port=2
  T6_in : Inport  Port=3
  m_dot_core : Inport  Port=4
  Const_DoUpgrade : Constant  Value=DoUpgrade  SampleTime=-1
  Discrete Transfer Fcn1 : DiscreteTransferFcn  Numerator=0.0031  Denominator=1 -0.9969  InitialStates=0.001
  Display{1..4} (4 alike) : DisplayBlock  LabelPosition=Hide  Transparency=1  GridColor=[0.502, 0.502, 0.502]
  Gain : Gain  Gain=Eff_Mod_LPT
  LPC_Upgraded : Constant  Value=Eff_Mod_LPC_Up
  LPT_Eff_LUT : Lookup_n-D  BreakpointsForDimension1=speed_vec_lpt  BreakpointsForDimension2=Wc_lpt_bp  Table=eta_lpt_map  ExtrapMethod=Clip  InternalRulePriority=Speed  RndMeth=Simplest
      settings: InputPortMap=u0,u1
  LPT_PR_LUT : Lookup_n-D  BreakpointsForDimension1=speed_vec_lpt  BreakpointsForDimension2=Wc_lpt_bp  Table=PR_lpt_map  ExtrapMethod=Clip  InternalRulePriority=Speed  RndMeth=Simplest
      settings: InputPortMap=u0,u1
  MATLAB Function : MATLAB Function  TreatAsAtomicUnit=on
  Memory : Memory
  Random Number : RandomNumber  Variance=0.5  SampleTime=0.001
  Sum : Sum  Inputs=|++
  Switch : Switch  Criteria=u2 > Threshold  Threshold=0.5  SaturateOnIntegerOverflow=off  InputSameDT=off
  flow_guess_LPT : Constant  Value=100
  T7_out : Outport
  P7_out : Outport  Port=2
  Torque_LPT : Outport  Port=3
  wires:
  Const_DoUpgrade/1 -> Switch/3
  MATLAB Function/1(P7_out) -> P7_out/1
  omega_N1/1 -> Memory/1
  LPC_Upgraded/1 -> Switch/2
  T6_in/1 -> MATLAB Function/2(T6_in)
  Gain/1 -> Switch/1  "eta_LPC"
  flow_guess_LPT/1 -> LPT_Eff_LUT/2, LPT_PR_LUT/2
  Memory/1 -> LPT_PR_LUT/1, LPT_Eff_LUT/1, MATLAB Function/5(N1_RPM)
  LPT_Eff_LUT/1 -> Gain/1
  LPT_PR_LUT/1 -> MATLAB Function/3(PR_LPT)
  Random Number/1 -> Discrete Transfer Fcn1/1
  P6_in/1 -> MATLAB Function/1(P6_in)
  Switch/1 -> MATLAB Function/4(eta_LPT)
  MATLAB Function/3(Torque_LPT) -> Torque_LPT/1
  m_dot_core/1 -> MATLAB Function/6(m_dot_core)
  Discrete Transfer Fcn1/1 -> Sum/1
  MATLAB Function/2(T7_out) -> Sum/2
  Sum/1 -> T7_out/1

== system TopLevel_Turbofan_DT_Faults/MissionPhaseIdentifier ==
  altitude : Inport
  throttle : Inport  Port=2
  MATLAB Function : MATLAB Function  TreatAsAtomicUnit=on
  Mission_Phase : Outport
  wires:
  MATLAB Function/1(phase) -> Mission_Phase/1
  throttle/1 -> MATLAB Function/2(throttle)
  altitude/1 -> MATLAB Function/1(altitude)

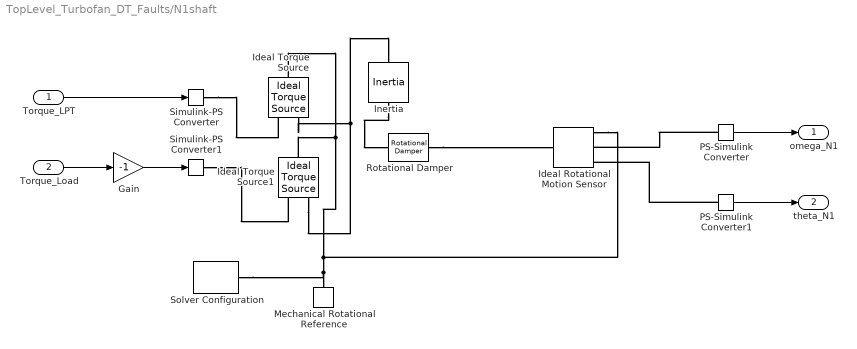
== system TopLevel_Turbofan_DT_Faults/N1shaft ==
  Torque_LPT : Inport
  Torque_Load : Inport  Port=2
  Gain : Gain  Gain=-1
  Ideal Rotational Motion Sensor : fl_lib/Mechanical/Mechanical Sensors/Ideal Rotational Motion Sensor  reference=foundation.enum.MeasurementReference.difference  acceleration_port=false  velocity_port=true  position_port=true  wrap_angle=false  offset=0 rad
      settings: LogSimulationData=on
  Ideal Torque Source : fl_lib/Mechanical/Mechanical Sources/Ideal Torque Source
  Ideal Torque Source1 : fl_lib/Mechanical/Mechanical Sources/Ideal Torque Source
  Inertia : fl_lib/Mechanical/Rotational Elements/Inertia  inertia=100 kg*m^2  num_ports=foundation.enum.numPorts2.two  w_specify=off  w_priority=High  w=52.36 rad/s  w_nominal_specify=off  w_nominal_value=1  w_nominal_unit=rad/s  t_specify=off  t_priority=None  t=0 N*m  t_nominal_specify=off  t_nominal_value=1  t_nominal_unit=N*m
      settings: InternalSimscapePortConfiguration="{\"Bottom\":[],\"Left\":[{\"id\":\"I\",\"label\":\"\",\"type\":\"foundation.mechanical.rotational.rotational\"}],\"Right\":[{\"id\":\"J\",\"label\":\"\",\"type\":\"foundation.mechanical.rotational.rotational\"}],\"Top\":[]}"
  Mechanical Rotational Reference : fl_lib/Mechanical/Rotational Elements/Mechanical Rotational Reference
  PS-Simulink Converter : nesl_utility/PS-Simulink Converter  PhysicalDomain=network_engine_domain  SubClassName=ps_output  LeftPortType=input  RightPortType=output  PseudoPeriodic=off  Frequencies=[]  VectorFormat=inherit  Unit=rad/s  AffineConversion=off
  PS-Simulink Converter1 : nesl_utility/PS-Simulink Converter  PhysicalDomain=network_engine_domain  SubClassName=ps_output  LeftPortType=input  RightPortType=output  PseudoPeriodic=off  Frequencies=[]  VectorFormat=inherit  Unit=rad  AffineConversion=off
  Rotational Damper : sdl_lib/Couplings & Drives/Springs & Dampers/Rotational Damper  D=10 N*m*s/rad  thermal_port=simscape.enum.thermaleffects.omit  thermal_mass=50 kJ/K  temperature_specify=off  temperature_priority=High  temperature=300 K  temperature_nominal_specify=off  temperature_nominal_value=1  temperature_nominal_unit=K
  Simulink-PS Converter : nesl_utility/Simulink-PS Converter  PhysicalDomain=network_engine_domain  SubClassName=ps_input  LeftPortType=input  RightPortType=output  PseudoPeriodic=off  Frequencies=[]  NoiseDistribution=none  NoiseParameters=[]  Unit=N*m  AffineConversion=off  FilteringAndDerivatives=provide  SimscapeFilterOrder=1  InputFilterTimeConstant=0.001  UdotUserProvided=0
  Simulink-PS Converter1 : nesl_utility/Simulink-PS Converter  PhysicalDomain=network_engine_domain  SubClassName=ps_input  LeftPortType=input  RightPortType=output  PseudoPeriodic=off  Frequencies=[]  NoiseDistribution=none  NoiseParameters=[]  Unit=N*m  AffineConversion=off  FilteringAndDerivatives=provide  SimscapeFilterOrder=1  InputFilterTimeConstant=0.001  UdotUserProvided=0
  Solver Configuration : nesl_utility/Solver Configuration  PhysicalDomain=network_engine_domain  SubClassName=solver  LeftPortType=input  RightPortType=generic  Tones=[]  Harmonics=[]  SimulateNoise=off  Profile=off  UseLocalSampling=off  EnableSwitchedLinearOptims=on  FrequencyDomain=off  UseCCode=off  RelTol=0.001  AbsTol=0.001  MinStep=1e-09  ToWorkspace=off  RevertToSquareIcSolve=off  NumHomotopyIterations=100  PhasorMode=off  PhasorModeNumHarmonics=1  ConsistencySolver=NEWTON_XTOL_AFTER_FTOL  IndexReductionMethod=DerivativeReplacement  DoDC=off  ResidualTolerance=1e-09  ConsistencyTolSource=GLOBAL  ConsistencyAbsTol=0.001  ConsistencyRelTol=0.001  ConsistencyTolFactor=0.001  UseLocalSolver=off  LocalSolverChoice=NE_BACKWARD_EULER_ADVANCER  ResolveIndetEquations=on  FunctionEvalNumThread=1  LocalSolverSampleTime=0.001  DoFixedCost=off  MaxNonlinIter=3  MaxModeIter=2  ComputeImpulses=off  ImpulseIterations=2  LinearAlgebra=auto  LinearAlgebraNumThread=0  EquationFormulation=NE_TIME_EF  DelaysMemoryBudget=1024  AutomaticFiltering=on  FilteringTimeConstant=0.001  PartitionStorageMethod=AS_NEEDED  PartitionMemoryBudget=1024  PartitionMethod=ROBUST  MultibodyUseLocalSolver=off  MultibodyLocalSolverChoice=ODE1  MultibodyLocalSolverSampleTime=0.001
  omega_N1 : Outport
  theta_N1 : Outport  Port=2
  wires:
  PS-Simulink Converter1/1 -> theta_N1/1
  PS-Simulink Converter/1 -> omega_N1/1
  Torque_LPT/1 -> Simulink-PS Converter/1
  Torque_Load/1 -> Gain/1
  Gain/1 -> Simulink-PS Converter1/1
  connections:
  Ideal Rotational Motion Sensor/RConn1 -- Ideal Torque Source/LConn1 -- Ideal Torque Source1/LConn1 -- Solver Configuration/RConn1 -- Mechanical Rotational Reference/LConn1
  Rotational Damper/RConn1 -- Ideal Rotational Motion Sensor/LConn1
  Inertia/RConn1 -- Rotational Damper/LConn1
  PS-Simulink Converter/LConn1 -- Ideal Rotational Motion Sensor/RConn2
  PS-Simulink Converter1/LConn1 -- Ideal Rotational Motion Sensor/RConn3
  Simulink-PS Converter1/RConn1 -- Ideal Torque Source1/RConn1
  Simulink-PS Converter/RConn1 -- Ideal Torque Source/RConn1
  Ideal Torque Source/RConn2 -- Ideal Torque Source1/RConn2 -- Inertia/LConn1

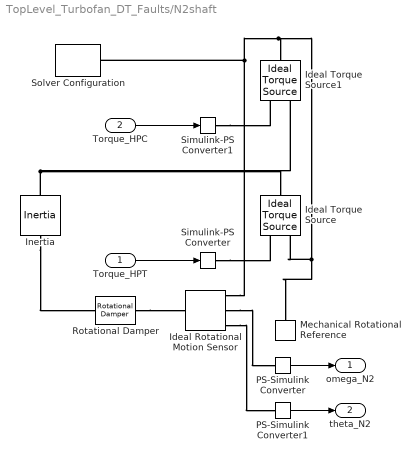
== system TopLevel_Turbofan_DT_Faults/N2shaft ==
  Torque_HPT : Inport
  Torque_HPC : Inport  Port=2
  Ideal Rotational Motion Sensor : fl_lib/Mechanical/Mechanical Sensors/Ideal Rotational Motion Sensor  reference=foundation.enum.MeasurementReference.difference  acceleration_port=false  velocity_port=true  position_port=true  wrap_angle=false  offset=0 rad
      settings: LogSimulationData=on
  Ideal Torque Source : fl_lib/Mechanical/Mechanical Sources/Ideal Torque Source
  Ideal Torque Source1 : fl_lib/Mechanical/Mechanical Sources/Ideal Torque Source
  Inertia : fl_lib/Mechanical/Rotational Elements/Inertia  inertia=2 kg*m^2  num_ports=foundation.enum.numPorts2.two  w_specify=on  w_priority=High  w=52.36 rad/s  w_nominal_specify=off  w_nominal_value=1  w_nominal_unit=rad/s  t_specify=off  t_priority=None  t=0 N*m  t_nominal_specify=off  t_nominal_value=1  t_nominal_unit=N*m
      settings: InternalSimscapePortConfiguration="{\"Bottom\":[],\"Left\":[{\"id\":\"I\",\"label\":\"\",\"type\":\"foundation.mechanical.rotational.rotational\"}],\"Right\":[{\"id\":\"J\",\"label\":\"\",\"type\":\"foundation.mechanical.rotational.rotational\"}],\"Top\":[]}"
  Mechanical Rotational Reference : fl_lib/Mechanical/Rotational Elements/Mechanical Rotational Reference
  PS-Simulink Converter : nesl_utility/PS-Simulink Converter  PhysicalDomain=network_engine_domain  SubClassName=ps_output  LeftPortType=input  RightPortType=output  PseudoPeriodic=off  Frequencies=[]  VectorFormat=inherit  Unit=rad/s  AffineConversion=off
  PS-Simulink Converter1 : nesl_utility/PS-Simulink Converter  PhysicalDomain=network_engine_domain  SubClassName=ps_output  LeftPortType=input  RightPortType=output  PseudoPeriodic=off  Frequencies=[]  VectorFormat=inherit  Unit=rad  AffineConversion=off
  Rotational Damper : sdl_lib/Couplings & Drives/Springs & Dampers/Rotational Damper  D=1 N*m*s/rad  thermal_port=simscape.enum.thermaleffects.omit  thermal_mass=50 kJ/K  temperature_specify=off  temperature_priority=High  temperature=300 K  temperature_nominal_specify=off  temperature_nominal_value=1  temperature_nominal_unit=K
  Simulink-PS Converter : nesl_utility/Simulink-PS Converter  PhysicalDomain=network_engine_domain  SubClassName=ps_input  LeftPortType=input  RightPortType=output  PseudoPeriodic=off  Frequencies=[]  NoiseDistribution=none  NoiseParameters=[]  Unit=N*m  AffineConversion=off  FilteringAndDerivatives=provide  SimscapeFilterOrder=1  InputFilterTimeConstant=0.001  UdotUserProvided=0
  Simulink-PS Converter1 : nesl_utility/Simulink-PS Converter  PhysicalDomain=network_engine_domain  SubClassName=ps_input  LeftPortType=input  RightPortType=output  PseudoPeriodic=off  Frequencies=[]  NoiseDistribution=none  NoiseParameters=[]  Unit=N*m  AffineConversion=off  FilteringAndDerivatives=provide  SimscapeFilterOrder=1  InputFilterTimeConstant=0.001  UdotUserProvided=0
  Solver Configuration : nesl_utility/Solver Configuration  PhysicalDomain=network_engine_domain  SubClassName=solver  LeftPortType=input  RightPortType=generic  Tones=[]  Harmonics=[]  SimulateNoise=off  Profile=off  UseLocalSampling=off  EnableSwitchedLinearOptims=on  FrequencyDomain=off  UseCCode=off  RelTol=0.001  AbsTol=0.001  MinStep=1e-09  ToWorkspace=off  RevertToSquareIcSolve=off  NumHomotopyIterations=100  PhasorMode=off  PhasorModeNumHarmonics=1  ConsistencySolver=NEWTON_XTOL_AFTER_FTOL  IndexReductionMethod=DerivativeReplacement  DoDC=off  ResidualTolerance=1e-09  ConsistencyTolSource=GLOBAL  ConsistencyAbsTol=0.001  ConsistencyRelTol=0.001  ConsistencyTolFactor=0.001  UseLocalSolver=off  LocalSolverChoice=NE_BACKWARD_EULER_ADVANCER  ResolveIndetEquations=on  FunctionEvalNumThread=1  LocalSolverSampleTime=0.001  DoFixedCost=off  MaxNonlinIter=3  MaxModeIter=2  ComputeImpulses=off  ImpulseIterations=2  LinearAlgebra=auto  LinearAlgebraNumThread=0  EquationFormulation=NE_TIME_EF  DelaysMemoryBudget=1024  AutomaticFiltering=on  FilteringTimeConstant=0.001  PartitionStorageMethod=AS_NEEDED  PartitionMemoryBudget=1024  PartitionMethod=ROBUST  MultibodyUseLocalSolver=off  MultibodyLocalSolverChoice=ODE1  MultibodyLocalSolverSampleTime=0.001
  omega_N2 : Outport
  theta_N2 : Outport  Port=2
  wires:
  Torque_HPT/1 -> Simulink-PS Converter/1
  Torque_HPC/1 -> Simulink-PS Converter1/1
  PS-Simulink Converter/1 -> omega_N2/1
  PS-Simulink Converter1/1 -> theta_N2/1
  connections:
  Simulink-PS Converter/RConn1 -- Ideal Torque Source/RConn1
  Inertia/RConn1 -- Rotational Damper/LConn1
  Ideal Rotational Motion Sensor/RConn1 -- Mechanical Rotational Reference/LConn1 -- Ideal Torque Source/RConn2 -- Ideal Torque Source1/LConn1 -- Solver Configuration/RConn1
  Simulink-PS Converter1/RConn1 -- Ideal Torque Source1/RConn1
  Rotational Damper/RConn1 -- Ideal Rotational Motion Sensor/LConn1
  Inertia/LConn1 -- Ideal Torque Source1/RConn2 -- Ideal Torque Source/LConn1
  Ideal Rotational Motion Sensor/RConn2 -- PS-Simulink Converter/LConn1
  Ideal Rotational Motion Sensor/RConn3 -- PS-Simulink Converter1/LConn1

== matlab function TopLevel_Turbofan_DT_Faults/HPC/CorrectedFlow ==
  data: P1 input; Wc output; T1 input
function Wc = Calc_Wc(P1, T1)
% Computes corrected mass flow [kg/s] from inlet total pressure and temperature

    % Constants
    Tref = 288.15;      % Reference temperature [K]
    Pref = 101325;      % Reference pressure [Pa]
    R = 287;            % J/(kg·K), gas constant for air
    A = 0.05;           % Inlet area [m^2]
    V = 100;            % Inlet velocity [m/s]

    % Safe Inputs
    T_safe = max(T1, eps);   % Avoid division by 0
    P_safe = max(P1, eps);   % Avoid division by 0

    % 1. Air density at inlet
    rho = P_safe / (R * T_safe);   % [kg/m^3]

    % 2. Actual mass flow
    m_dot = rho * A * V;           % [kg/s]

    % 3. Corrected mass flow
    temp_ratio = max(T_safe / Tref, eps);
    press_ratio = max(Pref / P_safe, eps);
    Wc = m_dot / sqrt(temp_ratio) * press_ratio;
end

== matlab function TopLevel_Turbofan_DT_Faults/HPC/HPC_Calculations ==
  data: P1 input; P2 output; T1 input; PR input; eta input; N2 input; T2 output; Torque_HPC output; Wc input
function [P2, T2, Torque_HPC] = HPC_CoreCalc(P1, T1, PR, eta, N2, Wc)
% Computes outlet pressure, temperature, and shaft torque for HPC
% Fully protected version for Simulink/Simscape compatibility

    % Constants
    gamma = 1.4;
    cp = 1004;
    Tref = 288.15;
    Pref = 101325;

    % Clamp all critical inputs to safe non-zero minimums
    P1_safe = max(P1, eps);
    T1_safe = max(T1, eps);
    PR_safe = max(PR, eps);
    eta_safe = max(eta, eps);
    omega = max(N2 * 2 * pi / 60, eps);  % rad/s

    % 1) Outlet pressure
    P2 = P1_safe * PR_safe;

    % 2) Outlet temperature using isentropic relation with efficiency
    T2 = T1_safe * (1 + (1 / eta_safe) * (PR_safe^((gamma - 1) / gamma) - 1));

    % 3) Actual mass flow from corrected flow
    temp_ratio = max(T1_safe / Tref, eps);
    press_ratio = max(P1_safe / Pref, eps);
    m_dot = Wc * sqrt(temp_ratio) * press_ratio;

    % 4) Enthalpy rise
    delta_h = cp * (T2 - T1_safe);

    % 5) Torque on N2 shaft
    torque_raw = (m_dot * delta_h) / omega;

    % 6) Final torque clamp to avoid inf/nan
    Torque_HPC = min(max(torque_raw, -1e6), 1e6);
end

== matlab function TopLevel_Turbofan_DT_Faults/FanNozzle/ComputeCoreThrust ==
  data: T1_fan input; Thrust output; m_dot_bypass input
function Thrust = ComputeFanThrust(T1_fan, m_dot_bypass)
    cp = 1004;             % J/kg·K (air)
    T_ambient = 288;       % K
    V_ambient = 0;         % m/s, stationary aircraft

    if T1_fan > T_ambient
        V_exit = sqrt(2 * cp * (T1_fan - T_ambient));
    else
        V_exit = 0;
    end

    Thrust = m_dot_bypass * (V_exit - V_ambient);
end

== matlab function TopLevel_Turbofan_DT_Faults/CoreNozzle/ComputeCoreThrust ==
  data: T7_in input; Thrust output; m_dot_core input
function Thrust = ComputeCoreThrust(T7_in, m_dot_core)
    cp = 1150;           % J/kg·K (core gas specific heat)
    T_ambient = 288;     % K (standard sea level)
    V_ambient = 0;       % m/s (static case)
    
    % Ensure physical realism
    if T7_in > T_ambient
        V_exit = sqrt(2 * cp * (T7_in - T_ambient));
    else
        V_exit = 0;
    end

    Thrust = m_dot_core * (V_exit - V_ambient);
end

== matlab function TopLevel_Turbofan_DT_Faults/MissionPhaseIdentifier/MATLAB Function ==
  data: altitude input; phase output; throttle input
function phase = DeterminePhase(altitude, throttle)
% Returns string mission phase:
% 'Takeoff', 'Climb', 'Cruise', 'Descent', 'Landing'

if throttle > 0.9 && altitude < 1000
    phase = "Takeoff";
elseif throttle > 0.7 && altitude < 9000
    phase = "Climb";
elseif throttle >= 0.5 && altitude >= 9000
    phase = "Cruise";
elseif throttle < 0.6 && altitude < 9000 && altitude > 500
    phase = "Descent";
elseif throttle < 0.4 && altitude <= 500
    phase = "Landing";
else
    phase = "Undefined";
end

== matlab function TopLevel_Turbofan_DT_Faults/FMS/AtmosphereModel ==
  data: Altitude input; P0 output; T0 output
function [P0, T0] = AtmosphereModel(Altitude)
% Calculates ambient pressure (P0) and temperature (T0) using ISA model

    T0_sea = 288.15;   % Sea level temperature (K)
    P0_sea = 101325;   % Sea level pressure (Pa)
    L = 0.0065;        % Lapse rate (K/m)
    R = 287.05;        % Gas constant (J/kg·K)
    g = 9.80665;       % Gravity (m/s²)

    if Altitude < 11000
        T0 = T0_sea - L * Altitude;
        P0 = P0_sea * (1 - (L * Altitude) / T0_sea)^(g / (R * L));
    else
        T0 = 216.65;
        P11 = P0_sea * (1 - (L * 11000) / T0_sea)^(g / (R * L));
        P0 = P11 * exp(-g * (Altitude - 11000) / (R * T0));
    end
end

== matlab function TopLevel_Turbofan_DT_Faults/CheckViability ==
  data: N1 input; status output; Thrust input; Fuel input
function status = CheckViability(N1, Thrust, Fuel)
%#codegen
  % Tunable thresholds
  MIN_N1     = 20000;   MAX_N1     = 30000;
  MIN_THRUST = 250000;  MAX_THRUST = 350000;
  MIN_FUEL   = 0.01;    MAX_FUEL   = 0.1;

  okN1     = (N1     >= MIN_N1)     && (N1     <= MAX_N1);
  okThrust = (Thrust >= MIN_THRUST) && (Thrust <= MAX_THRUST);
  okFuel   = (Fuel   >= MIN_FUEL)   && (Fuel   <= MAX_FUEL);

  if okN1 && okThrust && okFuel
    status = 1;
  else
    status = 0;
  end
end

== matlab function TopLevel_Turbofan_DT_Faults/LogStatus ==
  data: status input
function log(status)
assignin('base','FlightStatus', status);

== matlab function TopLevel_Turbofan_DT_Faults/Fan/Fan_CoreCalc ==
  data: P0_fan input; P1_fan output; T0_fan input; PR input; eta_fan input; N1 input; Wc_total input; BPR input; T1_fan_raw output; Torque_fan output; Wc_core output; m_dot_core output
function [P1_fan, T1_fan_raw, Torque_fan, Wc_core, m_dot_core] = Fan_CoreCalc( ...
          P0_fan, T0_fan, PR, eta_fan, N1, Wc_total, BPR)
% Master-level fan thermodynamics and torque with full guards

    % === CONSTANTS ===
    gamma = 1.4;
    cp = 1004;              % [J/(kg·K)]
    Tref = 288.15;          % [K]
    Pref = 101325;          % [Pa]

    % === INPUT SANITY GUARDS ===
    PR       = min(max(PR, 1.01), 2.5);        % Typical fan PR: 1.2–2.0
    eta_fan  = min(max(eta_fan, 0.3), 0.98);   % Reasonable range
    N1       = max(N1, 1e-3);                  % RPM ≥ 0.001
    P0_fan   = max(P0_fan, 50000);             % Prevent vacuum
    T0_fan   = max(T0_fan, 200);               % Prevent < -70°C
    Wc_total = max(Wc_total, 1e-3);            % ≥ 1 g/s
    BPR      = max(BPR, 0);                    % ≥ 0

    % === 1. Outlet Pressure ===
    P1_fan = P0_fan * PR;

    % === 2. Outlet Temperature ===
    T1_fan_raw = T0_fan * (1 + (1 / eta_fan) * (PR^((gamma - 1)/gamma) - 1));

    % === 3. Angular velocity (rad/s) ===
    omega1 = N1 * 2 * pi / 60;

    % === 4. Actual mass flow from corrected ===
    temp_ratio  = max(T0_fan / Tref, eps);
    press_ratio = max(P0_fan / Pref, eps);
    m_dot_total = Wc_total * sqrt(temp_ratio) * press_ratio;

    % === 5. Core vs bypass flow ===
    m_dot_core = m_dot_total / (1 + BPR);

    % === 6. Output corrected core flow ===
    Wc_core = m_dot_core / sqrt(temp_ratio) * (Pref / P0_fan);

    % === 7. Enthalpy rise ===
    delta_T = max(T1_fan_raw - T0_fan, 0);   % Prevent negative ΔT
    delta_h = cp * delta_T;

    % === 8. Torque calculation ===
    raw_torque = (m_dot_total * delta_h) / omega1;

    % === 9. Clamp torque to safe range ===
    Torque_fan = min(max(raw_torque, -1e6), 1e6);  % ±1 MN·m max

    % === Optional Debug Print ===
    % fprintf('[FAN] N1 = %.2f RPM, PR = %.2f, η = %.2f, Torque = %.2f\n', ...
    %         N1, PR, eta_fan, Torque_fan);
end

== matlab function TopLevel_Turbofan_DT_Faults/Fan/Calc_Fan_Wc ==
  data: P0_fan input; Wc_total output; T0_fan input
function Wc_total = Calc_Fan_Wc(P0_fan, T0_fan)
% Return corrected total mass-flow (core + bypass) in kg/s.
% Fully guarded for Simulink/Simscape code-gen.

    % ----- constants ----------------------------------------------------
    Tref = 288.15;          % K
    Pref = 101325;          % Pa
    R    = 287;             % J/(kg·K)
    A    = 0.50;            % m^2   (fan face area)
    V    = 120;             % m/s   (inlet velocity estimate)

    % ----- protect inputs ----------------------------------------------
    P  = max(P0_fan,  1e-3);    % avoid /0
    T  = max(T0_fan,  1e-3);

    % ----- density & actual mass-flow ----------------------------------
    rho          = P / (R * T);               % kg/m^3
    m_dot_total  = rho * A * V;               % kg/s

    % ----- corrected flow ----------------------------------------------
    temp_ratio   = max(T / Tref, eps);
    press_ratio  = max(Pref / P, eps);
    Wc_total_raw = m_dot_total / sqrt(temp_ratio) * press_ratio;

    % ----- clamp to physically plausible range -------------------------
    Wc_total = min(max(Wc_total_raw, 10), 2000);   % kg/s
end

== matlab function TopLevel_Turbofan_DT_Faults/LPT/MATLAB Function ==
  data: P6_in input; T6_in input; P7_out output; PR_LPT input; eta_LPT input; N1_RPM input; T7_out output; Torque_LPT output; m_dot_core input
function [P7_out, T7_out, Torque_LPT] = ...
    LPT_CalcCore(P6_in, T6_in, PR_LPT, eta_LPT, N1_RPM, m_dot_core)

% ===== constants & guards ==============================================
gamma = 1.4;  cp = 1004;

P6  = max(P6_in,  1e-3);
T6  = max(T6_in,  1e-3);
PR  = max(min(PR_LPT,0.98),0.50);    % turbine PR ≤ 1
eta = max(eta_LPT, 1e-3);
rpm = max(N1_RPM,  1e-3);
md  = max(m_dot_core, 1e-3);

% ===== outlet P/T =======================================================
P7_out = P6 * PR;
T7_out = T6 * (1 - eta*(1 - PR^((gamma-1)/gamma)));

% ===== torque ===========================================================
omega      = rpm * 2*pi/60;            % rad/s
delta_h    = cp * max(T6 - T7_out, 0); % positive J/kg
torque_raw = (md * delta_h) / max(omega, eps);
Torque_LPT = torque_raw;
end
